simulink model "Simulation"  (R2022a)
settings: Solver=FixedStepAuto  StartTime=0.0  StopTime=10.0  FixedStep=0.001  RelTol=1e-3
libraries: commchan3 x1
settings Model: Creator=ahmcmillon  LastModifiedBy=ahmcmillon
settings DataIOCC: ReturnWorkspaceOutputs=off

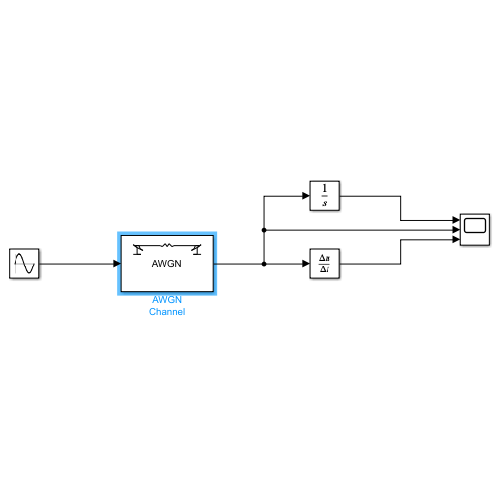
[thumbnail: Simulink's stored preview of the top-level diagram]
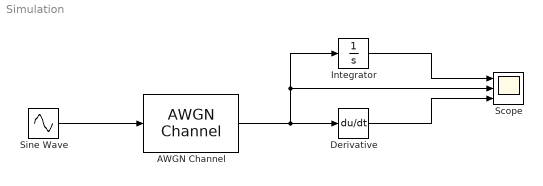
== system Simulation ==
  AWGN Channel : commchan3/AWGN Channel  InputProcessing=Columns as channels (frame based)  seed=67  noiseMode="Signal to noise ratio  (Eb/No)"  EbNodB=-20  EsNodB=10  SNRdB=10  bitsPerSym=1  Ps=1  Tsym=1  variance=1
  Derivative : Derivative
  Integrator : Integrator
  Scope : Scope  NumInputPorts=3
  Sine Wave : Sin  Amplitude=25  Frequency=5  SampleTime=0
  wires:
  Sine Wave/1 -> AWGN Channel/1
  AWGN Channel/1 -> Derivative/1, Integrator/1, Scope/2
  Integrator/1 -> Scope/1
  Derivative/1 -> Scope/3
